simulink model "TRN_KAISIM"  (R2022a)
settings: Solver=FixedStepAuto  StartTime=0.0  StopTime=300  FixedStep=0.04  RelTol=1e-3
PreLoadFcn:
  | load('BusStructureTRNsensor.mat');
  | load('BusStructureTRN.mat');
InitFcn:
  | load('BusStructureTRNsensor.mat');
  | load('BusStructureTRN.mat');
undefined symbols (not defined in the file or in its folder): Altitude_INS, Latitude_INS, Longitude_INS, residual, Result_Prev, TimeTag_Prev, TRN, TRNlib
libraries: simulink_extras x18, sharedtransform x3
(part 2 of 4)

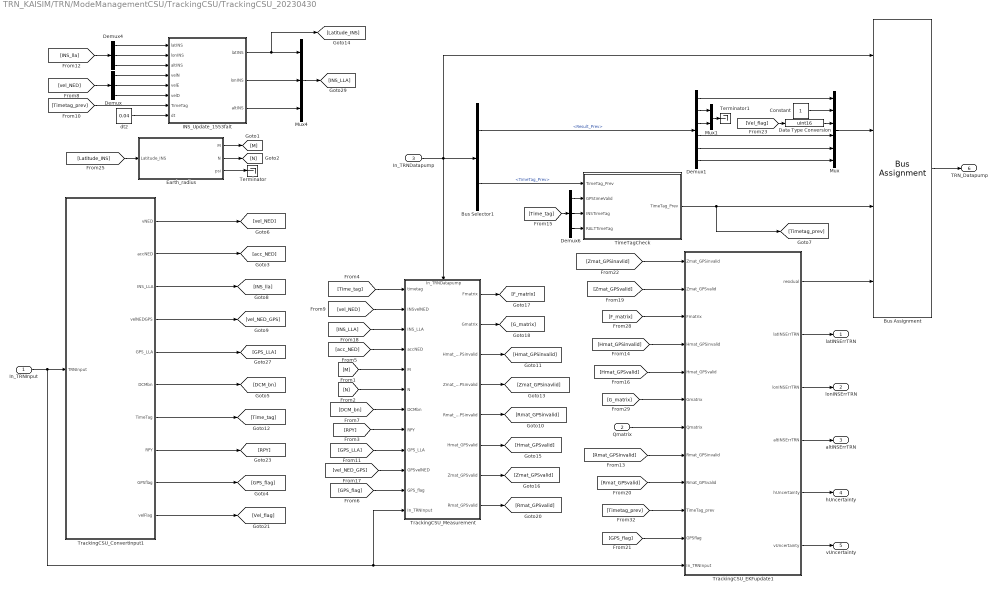
== system TRN_KAISIM/TRN/ModeManagementCSU/TrackingCSU/TrackingCSU_20230430 ==
  In_TRNInput : Inport  OutDataTypeStr=Bus: TRNInput
  Qmatrix : Inport  Port=2
  In_TRNDatapump : Inport  Port=3  OutDataTypeStr=Bus: TRNDatapump  PortDimensions=1
  Bus Assignment : BusAssignment  AssignedSignals=Result_Prev,TimeTag_Prev,residual
  Bus Selector1 : BusSelector  OutputSignals=Result_Prev,TimeTag_Prev
  Constant : Constant  OutDataTypeStr=uint16
  Data Type Conversion : DataTypeConversion  OutDataTypeStr=uint16  SaturateOnIntegerOverflow=off  RndMeth=Floor
  Demux : Demux  Outputs=3
  Demux1 : Demux  Outputs=6
  Demux4 : Demux  Outputs=3
  Demux6 : Demux  Outputs=3
  Earth_radius : MATLAB Function  TreatAsAtomicUnit=on
      settings: RTWSystemCode=Nonreusable function  RTWFcnNameOpts=Use subsystem name
  INS_Update_1553falt : MATLAB Function  TreatAsAtomicUnit=on
      settings: RTWSystemCode=Nonreusable function  RTWFcnNameOpts=Use subsystem name
  Mux : Mux  Inputs=6
  Mux1 : Mux  Inputs=2
  Mux4 : Mux  Inputs=3
  Terminator : Terminator
  Terminator1 : Terminator
  TimeTagCheck : MATLAB Function  TreatAsAtomicUnit=on
      settings: RTWSystemCode=Nonreusable function  RTWFcnNameOpts=Use subsystem name
  TrackingCSU_ConvertInput1 : Subsystem  TreatAsAtomicUnit=on
      settings: RTWSystemCode=Nonreusable function  RTWFcnNameOpts=Use subsystem name
  TrackingCSU_EKFupdate1 : Subsystem  TreatAsAtomicUnit=on
      settings: RTWSystemCode=Nonreusable function  RTWFcnNameOpts=Use subsystem name
  TrackingCSU_Measurement : Subsystem  TreatAsAtomicUnit=on
      settings: RTWSystemCode=Nonreusable function  RTWFcnNameOpts=Use subsystem name  PortSchema="{\"entries\":[{\"content\":{\"sides\":[{\"content\":{\"connectorIds\":[\"In1\",\"In2\",\"In3\",\"In4\",\"In5\",\"In6\",\"In7\",\"In8\",\"In9\",\"In10\",\"In11\",\"In12\"]},\"type\":\"ConnectorPlacement.EquallySpacedRectSide\",\"uuid\":\"284c5e42-61c1-4616-966e-143f60f46571\"},{\"content\":{\"connectorIds\":[\"Out1\",\"Out2\",\"Out3\",\"Out4\",\"Out5\",\"Out6\",\"Out7\",\"Out8\"],\"side\":\"RIGHT\"},\"type\":\"ConnectorPlacement.EquallySpacedRectSide\",\"uuid\":\"be5b0b09-4e69-4cdf-8a94-a8639994cbf9\"},{\"content\":{\"connectorIds\":[\"In13\"],\"side\":\"TOP\"},\"type\":\"ConnectorPlacement.EquallySpacedRectSide\",\"uuid\":\"f7fbee8b-afe7-4fec-8c40-a5bd5e14374e\"},{\"content\":{\"connectorIds\":[],\"side\":\"BOTTOM\"},\"type\":\"ConnectorPlacement.EquallySpacedRectSide\",\"uuid\":\"9a503e43-aaca-441a-ab76-b52386228bc3\"}]},\"type\":\"ConnectorPlacement.EquallySpacedConnector\",\"uuid\":\"1b32203e-baad-4c49-8c24-20b6a9ecb4b9\"}],\"packageUris\":[\"http://schema.mathworks.com/mf0/Connector/R2020b\"],\"version\":\"1.0\"}"
  dt2 : Constant  Value=0.04  OutDataTypeStr=double
  latINSErrTRN : Outport
  lonINSErrTRN : Outport  Port=2
  altINSErrTRN : Outport  Port=3
  hUncertainty : Outport  Port=4
  vUncertainty : Outport  Port=5
  TRN_Datapump : Outport  Port=6  OutDataTypeStr=Bus: TRNDatapump
  wires:
  Mux4/1 -> [INS_LLA]
  Demux/3 -> INS_Update_1553falt/6(velD)
  Demux/1 -> INS_Update_1553falt/4(velN)
  Demux/2 -> INS_Update_1553falt/5(velE)
  dt2/1 -> INS_Update_1553falt/8(dt)
  Bus Selector1/2 -> TimeTagCheck/1("TimeTag_Prev ")  "<TimeTag_Prev>"
  In_TRNDatapump/1 -> TrackingCSU_Measurement/13(In_TRNDatapump), Bus Selector1/1, Bus Assignment/1
  INS_Update_1553falt/3(altINS) -> Mux4/3
  In_TRNInput/1 -> TrackingCSU_ConvertInput1/1(TRNInput), TrackingCSU_EKFupdate1/12(In_TRNInput), TrackingCSU_Measurement/12(In_TRNInput)
  INS_Update_1553falt/1(latINS) -> [Latitude_INS], Mux4/1
  INS_Update_1553falt/2(lonINS) -> Mux4/2
  TrackingCSU_ConvertInput1/2(accNED) -> [acc_NED]
  TrackingCSU_ConvertInput1/6(DCMbn) -> [DCM_bn]
  TrackingCSU_ConvertInput1/1(vNED) -> [vel_NED]
  [vel_NED] -> Demux/1
  [Timetag_prev] -> INS_Update_1553falt/7(TimeTag)
  [INS_lla] -> Demux4/1
  Demux4/2 -> INS_Update_1553falt/2("lonINS ")
  Demux4/1 -> INS_Update_1553falt/1("latINS ")
  Demux4/3 -> INS_Update_1553falt/3("altINS ")
  TrackingCSU_ConvertInput1/4(velNEDGPS) -> [vel_NED_GPS]
  [Time_tag] -> Demux6/1
  Demux6/1 -> TimeTagCheck/2(GPStimeValid)
  Demux6/2 -> TimeTagCheck/3(INSTimeTag)
  Demux6/3 -> TimeTagCheck/4(RALTTimeTag)
  TrackingCSU_Measurement/1(Fmatrix) -> [F_matrix]
  TrackingCSU_Measurement/2(Gmatrix) -> [G_matrix]
  [Zmat_GPSinavlid] -> TrackingCSU_EKFupdate1/1(Zmat_GPSinvalid)
  [Latitude_INS] -> Earth_radius/1(Latitude_INS)
  Earth_radius/1(M) -> [M]
  Earth_radius/2(N) -> [N]
  TrackingCSU_ConvertInput1/5(GPS_LLA) -> [GPS_LLA]
  TrackingCSU_ConvertInput1/8(RPY) -> [RPY]
  TimeTagCheck/1(TimeTag_Prev) -> [Timetag_prev], Bus Assignment/3
  TrackingCSU_ConvertInput1/9(GPSflag) -> [GPS_flag]
  TrackingCSU_ConvertInput1/7(TimeTag) -> [Time_tag]
  TrackingCSU_ConvertInput1/3(INS_LLA) -> [INS_lla]
  Earth_radius/3(psi) -> Terminator/1
  TrackingCSU_Measurement/3(Hmat_GPSinvalid) -> [Hmat_GPSinvalid]
  TrackingCSU_Measurement/4(Zmat_GPSinvalid) -> [Zmat_GPSinavlid]
  TrackingCSU_Measurement/5(Rmat_GPSinvalid) -> [Rmat_GPSinvalid]
  TrackingCSU_Measurement/6(Hmat_GPSvalid) -> [Hmat_GPSvalid]
  TrackingCSU_Measurement/7(Zmat_GPSvalid) -> [Zmat_GPSvalid]
  TrackingCSU_Measurement/8(Rmat_GPSvalid) -> [Rmat_GPSvalid]
  [GPS_flag] -> TrackingCSU_EKFupdate1/11(GPSflag)
  [Rmat_GPSvalid] -> TrackingCSU_EKFupdate1/9(Rmat_GPSvalid)
  [Rmat_GPSinvalid] -> TrackingCSU_EKFupdate1/8(Rmat_GPSinvalid)
  Qmatrix/1 -> TrackingCSU_EKFupdate1/7(Qmatrix)
  [G_matrix] -> TrackingCSU_EKFupdate1/6(Gmatrix)
  [Hmat_GPSvalid] -> TrackingCSU_EKFupdate1/5(Hmat_GPSvalid)
  [Hmat_GPSinvalid] -> TrackingCSU_EKFupdate1/4(Hmat_GPSinvalid)
  [F_matrix] -> TrackingCSU_EKFupdate1/3(Fmatrix)
  [Zmat_GPSvalid] -> TrackingCSU_EKFupdate1/2(Zmat_GPSvalid)
  TrackingCSU_EKFupdate1/2(latINSErrTRN) -> latINSErrTRN/1
  TrackingCSU_EKFupdate1/3(lonINSErrTRN) -> lonINSErrTRN/1
  TrackingCSU_EKFupdate1/4(altINSErrTRN) -> altINSErrTRN/1
  TrackingCSU_EKFupdate1/5(hUncertainty) -> hUncertainty/1
  TrackingCSU_EKFupdate1/6(vUncertainty) -> vUncertainty/1
  [Timetag_prev] -> TrackingCSU_EKFupdate1/10(TimeTag_prev)
  [GPS_LLA] -> TrackingCSU_Measurement/9(GPS_LLA)
  [vel_NED_GPS] -> TrackingCSU_Measurement/10(GPSvelNED)
  [GPS_flag] -> TrackingCSU_Measurement/11(GPS_flag)
  [Time_tag] -> TrackingCSU_Measurement/1(timetag)
  [INS_LLA] -> TrackingCSU_Measurement/3(INS_LLA)
  [acc_NED] -> TrackingCSU_Measurement/4(accNED)
  [DCM_bn] -> TrackingCSU_Measurement/7(DCMbn)
  [RPY] -> TrackingCSU_Measurement/8(RPY)
  [M] -> TrackingCSU_Measurement/5(M)
  [N] -> TrackingCSU_Measurement/6(N)
  [vel_NED] -> TrackingCSU_Measurement/2(INSvelNED)
  Bus Assignment/1 -> TRN_Datapump/1
  Mux/1 -> Bus Assignment/2
  Demux1/1 -> Mux/1
  Demux1/5 -> Mux/5
  Demux1/6 -> Mux/6
  TrackingCSU_ConvertInput1/10(velFlag) -> [Vel_flag]
  [Vel_flag] -> Data Type Conversion/1
  Data Type Conversion/1 -> Mux/3
  Constant/1 -> Mux/2
  Demux1/4 -> Mux/4
  Demux1/3 -> Mux1/2
  Demux1/2 -> Mux1/1
  Mux1/1 -> Terminator1/1
  Bus Selector1/1 -> Demux1/1  "<Result_Prev>"
  TrackingCSU_EKFupdate1/1(residual) -> Bus Assignment/4

== system TRN_KAISIM/TRN/TRN_visualization/Subsystem ==
  In1 : Inport
  In2 : Inport  Port=2
  In3 : Inport  Port=3
  In4 : Inport  Port=4
  In5 : Inport  Port=5
  In6 : Inport  Port=6
  Gain2 : Gain  Gain=111000
  Gain3 : Gain  Gain=91170
  MATLAB Function1 : MATLAB Function  TreatAsAtomicUnit=on
  Sum : Sum  Inputs=|+-
  Sum1 : Sum  Inputs=|+-
  Sum2 : Sum  Inputs=|+-
  Terrain_Level_big4 : MATLAB Function  TreatAsAtomicUnit=on
  TRN Position Error Horizon : Outport
  TRN Position Error Vertical : Outport  Port=2
  Roughness : Outport  Port=3
  wires:
  Sum1/1 -> Gain3/1
  In1/1 -> Terrain_Level_big4/1(Lat), Sum/1
  In3/1 -> Terrain_Level_big4/2(Lon), Sum1/1
  Terrain_Level_big4/1(R) -> Roughness/1
  Gain2/1 -> MATLAB Function1/1(y)  "LatErr"
  Gain3/1 -> MATLAB Function1/2(x)  "LonErr"
  Sum2/1 -> TRN Position Error Vertical/1
  Sum/1 -> Gain2/1
  In4/1 -> Sum1/2
  In2/1 -> Sum/2
  In6/1 -> Sum2/2
  In5/1 -> Sum2/1
  MATLAB Function1/1(a) -> TRN Position Error Horizon/1

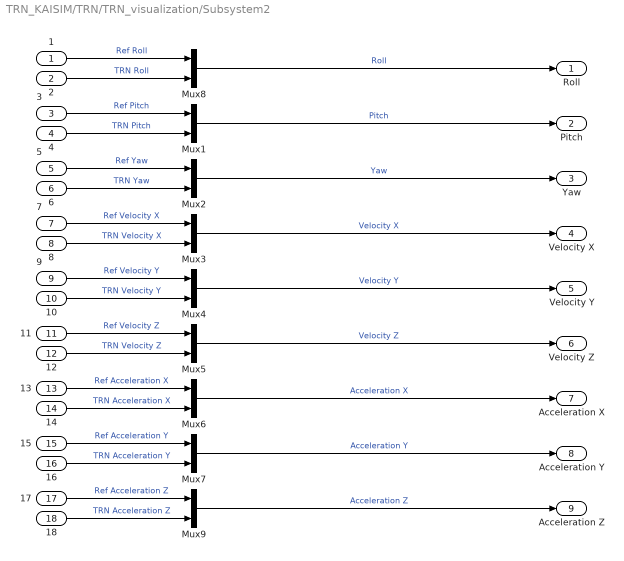
== system TRN_KAISIM/TRN/TRN_visualization/Subsystem2 ==
  1 : Inport
  2 : Inport  Port=2
  3 : Inport  Port=3
  4 : Inport  Port=4
  5 : Inport  Port=5
  6 : Inport  Port=6
  7 : Inport  Port=7
  8 : Inport  Port=8
  9 : Inport  Port=9
  10 : Inport  Port=10
  11 : Inport  Port=11
  12 : Inport  Port=12
  13 : Inport  Port=13
  14 : Inport  Port=14
  15 : Inport  Port=15
  16 : Inport  Port=16
  17 : Inport  Port=17
  18 : Inport  Port=18
  Mux{1..9} (9 alike) : Mux  Inputs=2
  Roll : Outport
  Pitch : Outport  Port=2
  Yaw : Outport  Port=3
  Velocity X : Outport  Port=4
  Velocity Y : Outport  Port=5
  Velocity Z : Outport  Port=6
  Acceleration X : Outport  Port=7
  Acceleration Y : Outport  Port=8
  Acceleration Z : Outport  Port=9
  wires:
  3/1 -> Mux1/1  "Ref Pitch"
  12/1 -> Mux5/2  "TRN Velocity Z"
  10/1 -> Mux4/2  "TRN Velocity Y"
  Mux9/1 -> Acceleration Z/1  "Acceleration Z"
  Mux8/1 -> Roll/1  "Roll"
  9/1 -> Mux4/1  "Ref Velocity Y"
  8/1 -> Mux3/2  "TRN Velocity X"
  5/1 -> Mux2/1  "Ref Yaw"
  Mux4/1 -> Velocity Y/1  "Velocity Y"
  1/1 -> Mux8/1  "Ref Roll"
  Mux6/1 -> Acceleration X/1  "Acceleration X"
  Mux7/1 -> Acceleration Y/1  "Acceleration Y"
  4/1 -> Mux1/2  "TRN Pitch"
  11/1 -> Mux5/1  "Ref Velocity Z"
  16/1 -> Mux7/2  "TRN Acceleration Y"
  Mux3/1 -> Velocity X/1  "Velocity X"
  Mux2/1 -> Yaw/1  "Yaw"
  2/1 -> Mux8/2  "TRN Roll"
  6/1 -> Mux2/2  "TRN Yaw"
  7/1 -> Mux3/1  "Ref Velocity X"
  Mux5/1 -> Velocity Z/1  "Velocity Z"
  Mux1/1 -> Pitch/1  "Pitch"
  15/1 -> Mux7/1  "Ref Acceleration Y"
  14/1 -> Mux6/2  "TRN Acceleration X"
  17/1 -> Mux9/1  "Ref Acceleration Z"
  18/1 -> Mux9/2  "TRN Acceleration Z"
  13/1 -> Mux6/1  "Ref Acceleration X"

== system TRN_KAISIM/TRN/TRN_visualization/Subsystem3 ==
  In1 : Inport
  In2 : Inport  Port=2
  In3 : Inport  Port=3
  In4 : Inport  Port=4
  In5 : Inport  Port=5
  In6 : Inport  Port=6
  Gain2 : Gain  Gain=111000
  Gain3 : Gain  Gain=91170
  MATLAB Function1 : MATLAB Function  TreatAsAtomicUnit=on
  Sum : Sum  Inputs=|+-
  Sum1 : Sum  Inputs=|+-
  Sum2 : Sum  Inputs=|+-
  Terrain_Level : MATLAB Function  TreatAsAtomicUnit=on
  TRN Position Error Horizon : Outport
  TRN Position Error Vertical : Outport  Port=2
  Roughness : Outport  Port=3
  wires:
  Sum1/1 -> Gain3/1
  In1/1 -> Terrain_Level/1(Lat), Sum/1
  In3/1 -> Terrain_Level/2(Lon), Sum1/1
  Terrain_Level/1(R) -> Roughness/1
  Gain2/1 -> MATLAB Function1/1(y)  "LatErr"
  Gain3/1 -> MATLAB Function1/2(x)  "LonErr"
  Sum2/1 -> TRN Position Error Vertical/1
  Sum/1 -> Gain2/1
  In4/1 -> Sum1/2
  In2/1 -> Sum/2
  In6/1 -> Sum2/2
  In5/1 -> Sum2/1
  MATLAB Function1/1(a) -> TRN Position Error Horizon/1

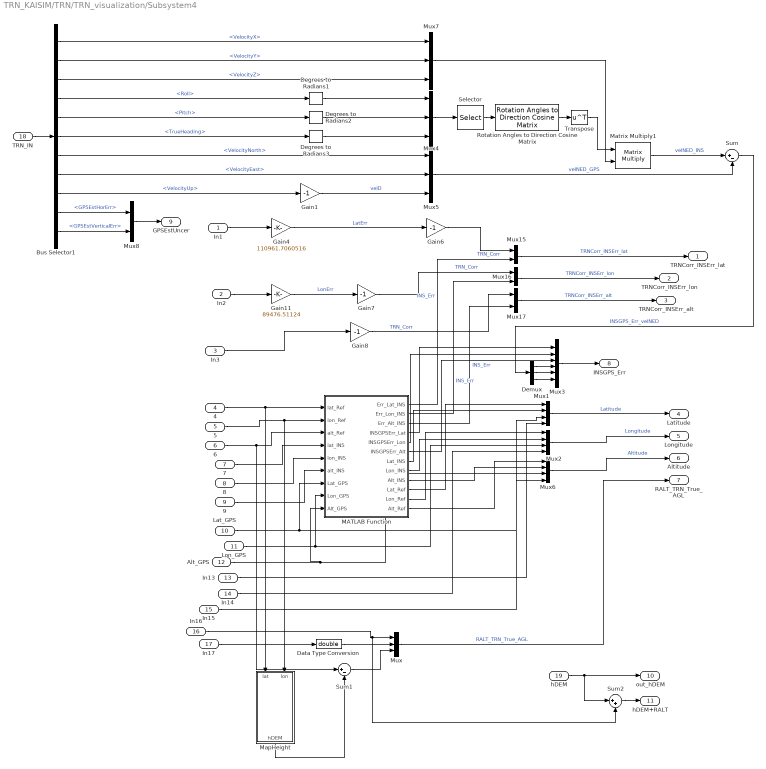
== system TRN_KAISIM/TRN/TRN_visualization/Subsystem4 ==
  In1 : Inport
  In2 : Inport  Port=2
  In3 : Inport  Port=3
  4 : Inport  Port=4
  5 : Inport  Port=5
  6 : Inport  Port=6
  7 : Inport  Port=7
  8 : Inport  Port=8
  9 : Inport  Port=9
  Lat_GPS : Inport  Port=10
  Lon_GPS : Inport  Port=11
  Alt_GPS : Inport  Port=12
  In13 : Inport  Port=13
  In14 : Inport  Port=14
  In15 : Inport  Port=15
  In16 : Inport  Port=16
  In17 : Inport  Port=17
  TRN_IN : Inport  Port=18
  hDEM : Inport  Port=19
  Bus Selector1 : BusSelector  OutputSignals=VelocityX,VelocityY,VelocityZ,Roll,Pitch,TrueHeading,VelocityNorth,VelocityEast,VelocityUp,GPSEstHorErr,GPSEstVerticalErr
  Data Type Conversion : DataTypeConversion  OutDataTypeStr=double  SaturateOnIntegerOverflow=off  RndMeth=Floor
  Degrees to Radians1 : simulink_extras/Transformations/Degrees to Radians
  Degrees to Radians2 : simulink_extras/Transformations/Degrees to Radians
  Degrees to Radians3 : simulink_extras/Transformations/Degrees to Radians
  Demux : Demux  Outputs=3
  Gain{1,6..8} (4 alike) : Gain  Gain=-1
  Gain11 : Gain  Gain=89476.51124
  Gain4 : Gain  Gain=110961.7060516
  MATLAB Function : MATLAB Function  TreatAsAtomicUnit=on
  MapHeight : MATLAB Function  TreatAsAtomicUnit=on
  Matrix Multiply1 : Product  Multiplication=Matrix(*)
  Mux{,4..5,7} (4 alike) : Mux  Inputs=3
  Mux1 : Mux
  Mux{8,15..17} (4 alike) : Mux  Inputs=2
  Mux2 : Mux
  Mux3 : Mux  Inputs=6
  Mux6 : Mux
  Rotation Angles to Direction Cosine Matrix : sharedtransform/Rotation Angles to Direction Cosine Matrix  rotationOrder=ZYX  aMode=aMode
      settings: SourceProductBaseCode=AE,PW,DR,MT,VE
  Selector : Selector  InputPortWidth=3  IndexOptions=Index vector (dialog)  Indices=[3 2 1]  OutputSizes=1
  Sum : Sum  Inputs=|+-
  Sum1 : Sum  Inputs=|+-
  Sum2 : Sum  Inputs=|++
  Transpose : Math  Operator=transpose  SignedPower=on
  TRNCorr_INSErr_lat : Outport
  TRNCorr_INSErr_lon : Outport  Port=2
  TRNCorr_INSErr_alt : Outport  Port=3
  Latitude : Outport  Port=4
  Longitude : Outport  Port=5
  Altitude : Outport  Port=6
  RALT_TRN_True_AGL : Outport  Port=7
  INSGPS_Err : Outport  Port=8
  GPSEstUncer : Outport  Port=9
  out_hDEM : Outport  Port=10
  hDEM+RALT : Outport  Port=11
  wires:
  7/1 -> MATLAB Function/4(lat_INS)
  MATLAB Function/10(Lat_Ref) -> Mux1/1
  Gain8/1 -> Mux17/1  "TRN_Corr"
  MATLAB Function/7(Lat_INS) -> Mux1/2
  MATLAB Function/8(Lon_INS) -> Mux2/2
  MATLAB Function/3(Err_Alt_INS) -> Mux17/2  "INS_Err"
  In13/1 -> Mux1/4
  Gain7/1 -> Mux16/1  "TRN_Corr"
  Mux1/1 -> Latitude/1  "Latitude"
  MATLAB Function/1(Err_Lat_INS) -> Mux15/2  "INS_Err"
  MATLAB Function/12(Alt_Ref) -> Mux6/1
  4/1 -> MapHeight/1(lat), MATLAB Function/1(lat_Ref)
  Gain11/1 -> Gain7/1  "LonErr"
  Gain6/1 -> Mux15/1  "TRN_Corr"
  MATLAB Function/9(Alt_INS) -> Mux6/2
  MATLAB Function/2(Err_Lon_INS) -> Mux16/2  "INS_Err"
  Mux17/1 -> TRNCorr_INSErr_alt/1  "TRNCorr_INSErr_alt"
  Gain4/1 -> Gain6/1  "LatErr"
  MATLAB Function/11(Lon_Ref) -> Mux2/1
  Lat_GPS/1 -> MATLAB Function/7(Lat_GPS), Mux1/3
  Mux2/1 -> Longitude/1  "Longitude"
  In3/1 -> Gain8/1
  Data Type Conversion/1 -> Mux/2
  8/1 -> MATLAB Function/5(lon_INS)
  Mux/1 -> RALT_TRN_True_AGL/1  "RALT_TRN_True_AGL"
  In17/1 -> Data Type Conversion/1
  9/1 -> MATLAB Function/6(alt_INS)
  Lon_GPS/1 -> MATLAB Function/8(Lon_GPS), Mux2/3
  Alt_GPS/1 -> MATLAB Function/9(Alt_GPS), Mux6/3
  In2/1 -> Gain11/1
  Mux16/1 -> TRNCorr_INSErr_lon/1  "TRNCorr_INSErr_lon"
  Mux6/1 -> Altitude/1  "Altitude"
  In1/1 -> Gain4/1
  In15/1 -> Mux6/4
  In14/1 -> Mux2/4
  6/1 -> Sum1/1, MATLAB Function/3(alt_Ref)
  5/1 -> MapHeight/2(lon), MATLAB Function/2(lon_Ref)
  Mux15/1 -> TRNCorr_INSErr_lat/1  "TRNCorr_INSErr_lat"
  MATLAB Function/5(INSGPSErr_Lon) -> Mux3/2
  MATLAB Function/4(INSGPSErr_Lat) -> Mux3/1
  MATLAB Function/6(INSGPSErr_Alt) -> Mux3/3
  Mux3/1 -> INSGPS_Err/1
  Mux7/1 -> Matrix Multiply1/2
  Degrees to Radians3/1 -> Mux4/3
  Degrees to Radians1/1 -> Mux4/1
  Bus Selector1/4 -> Degrees to Radians1/1  "<Roll>"
  Bus Selector1/6 -> Degrees to Radians3/1  "<TrueHeading>"
  Matrix Multiply1/1 -> Sum/1  "velNED_INS"
  Bus Selector1/5 -> Degrees to Radians2/1  "<Pitch>"
  Degrees to Radians2/1 -> Mux4/2
  Bus Selector1/2 -> Mux7/2  "<VelocityY>"
  Bus Selector1/1 -> Mux7/1  "<VelocityX>"
  Mux4/1 -> Selector/1
  Transpose/1 -> Matrix Multiply1/1
  Bus Selector1/3 -> Mux7/3  "<VelocityZ>"
  TRN_IN/1 -> Bus Selector1/1
  Rotation Angles to Direction Cosine Matrix/1 -> Transpose/1
  Selector/1 -> Rotation Angles to Direction Cosine Matrix/1
  Bus Selector1/7 -> Mux5/1  "<VelocityNorth>"
  Bus Selector1/8 -> Mux5/2  "<VelocityEast>"
  Bus Selector1/9 -> Gain1/1  "<VelocityUp>"
  Gain1/1 -> Mux5/3  "velD"
  Mux5/1 -> Sum/2  "velNED_GPS"
  Demux/1 -> Mux3/4
  Demux/2 -> Mux3/5
  Demux/3 -> Mux3/6
  Sum/1 -> Demux/1  "INSGPS_Err_velNED"
  Bus Selector1/10 -> Mux8/1  "<GPSEstHorErr>"
  Bus Selector1/11 -> Mux8/2  "<GPSEstVerticalErr>"
  Mux8/1 -> GPSEstUncer/1
  MapHeight/1(hDEM) -> Sum1/2
  Sum1/1 -> Mux/3
  In16/1 -> Sum2/2, Mux/1
  hDEM/1 -> out_hDEM/1, Sum2/1
  Sum2/1 -> hDEM+RALT/1

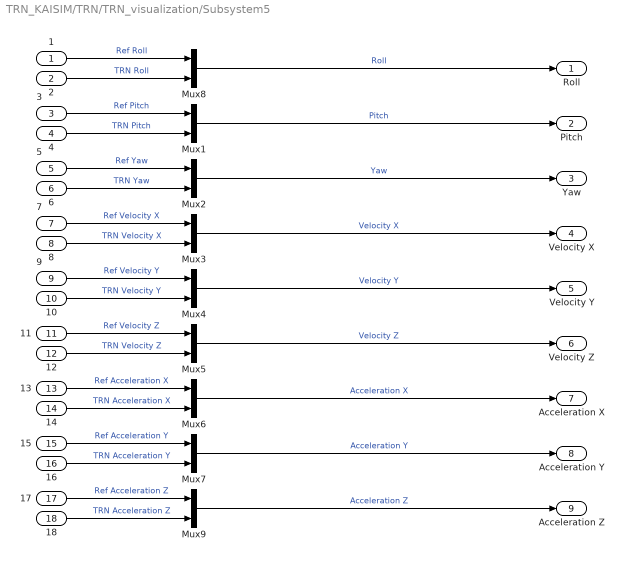
== system TRN_KAISIM/TRN/TRN_visualization/Subsystem5 ==
  1 : Inport
  2 : Inport  Port=2
  3 : Inport  Port=3
  4 : Inport  Port=4
  5 : Inport  Port=5
  6 : Inport  Port=6
  7 : Inport  Port=7
  8 : Inport  Port=8
  9 : Inport  Port=9
  10 : Inport  Port=10
  11 : Inport  Port=11
  12 : Inport  Port=12
  13 : Inport  Port=13
  14 : Inport  Port=14
  15 : Inport  Port=15
  16 : Inport  Port=16
  17 : Inport  Port=17
  18 : Inport  Port=18
  Mux{1..9} (9 alike) : Mux  Inputs=2
  Roll : Outport
  Pitch : Outport  Port=2
  Yaw : Outport  Port=3
  Velocity X : Outport  Port=4
  Velocity Y : Outport  Port=5
  Velocity Z : Outport  Port=6
  Acceleration X : Outport  Port=7
  Acceleration Y : Outport  Port=8
  Acceleration Z : Outport  Port=9
  wires:
  3/1 -> Mux1/1  "Ref Pitch"
  12/1 -> Mux5/2  "TRN Velocity Z"
  10/1 -> Mux4/2  "TRN Velocity Y"
  Mux9/1 -> Acceleration Z/1  "Acceleration Z"
  Mux8/1 -> Roll/1  "Roll"
  9/1 -> Mux4/1  "Ref Velocity Y"
  8/1 -> Mux3/2  "TRN Velocity X"
  5/1 -> Mux2/1  "Ref Yaw"
  Mux4/1 -> Velocity Y/1  "Velocity Y"
  1/1 -> Mux8/1  "Ref Roll"
  Mux6/1 -> Acceleration X/1  "Acceleration X"
  Mux7/1 -> Acceleration Y/1  "Acceleration Y"
  4/1 -> Mux1/2  "TRN Pitch"
  11/1 -> Mux5/1  "Ref Velocity Z"
  16/1 -> Mux7/2  "TRN Acceleration Y"
  Mux3/1 -> Velocity X/1  "Velocity X"
  Mux2/1 -> Yaw/1  "Yaw"
  2/1 -> Mux8/2  "TRN Roll"
  6/1 -> Mux2/2  "TRN Yaw"
  7/1 -> Mux3/1  "Ref Velocity X"
  Mux5/1 -> Velocity Z/1  "Velocity Z"
  Mux1/1 -> Pitch/1  "Pitch"
  15/1 -> Mux7/1  "Ref Acceleration Y"
  14/1 -> Mux6/2  "TRN Acceleration X"
  17/1 -> Mux9/1  "Ref Acceleration Z"
  18/1 -> Mux9/2  "TRN Acceleration Z"
  13/1 -> Mux6/1  "Ref Acceleration X"

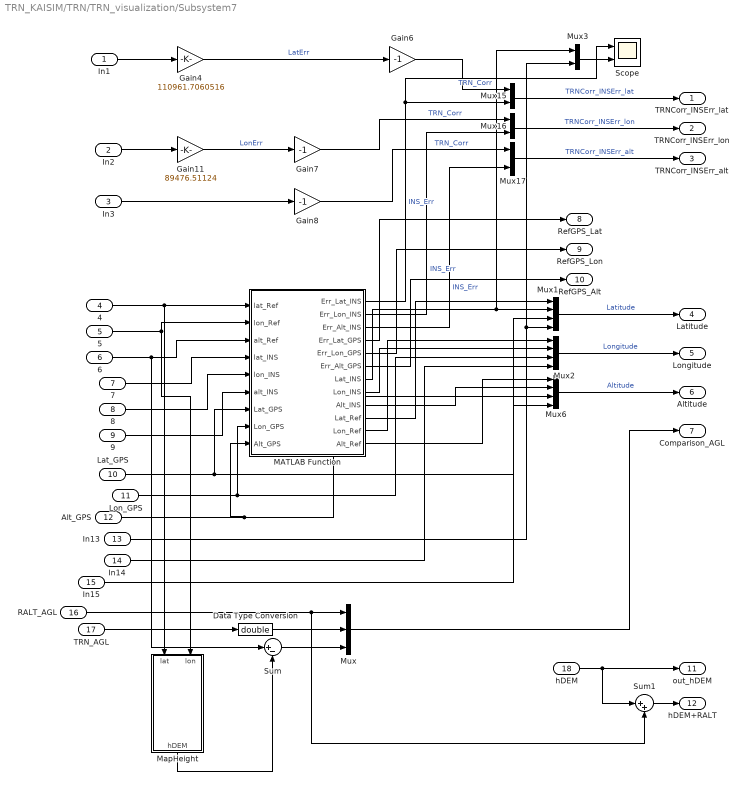
== system TRN_KAISIM/TRN/TRN_visualization/Subsystem7 ==
  In1 : Inport
  In2 : Inport  Port=2
  In3 : Inport  Port=3
  4 : Inport  Port=4
  5 : Inport  Port=5
  6 : Inport  Port=6
  7 : Inport  Port=7
  8 : Inport  Port=8
  9 : Inport  Port=9
  Lat_GPS : Inport  Port=10
  Lon_GPS : Inport  Port=11
  Alt_GPS : Inport  Port=12
  In13 : Inport  Port=13
  In14 : Inport  Port=14
  In15 : Inport  Port=15
  RALT_AGL : Inport  Port=16
  TRN_AGL : Inport  Port=17
  hDEM : Inport  Port=18
  Data Type Conversion : DataTypeConversion  OutDataTypeStr=double  SaturateOnIntegerOverflow=off  RndMeth=Floor
  Gain11 : Gain  Gain=89476.51124
  Gain4 : Gain  Gain=110961.7060516
  Gain6 : Gain  Gain=-1
  Gain7 : Gain  Gain=-1
  Gain8 : Gain  Gain=-1
  MATLAB Function : MATLAB Function  TreatAsAtomicUnit=on
  MapHeight : MATLAB Function  TreatAsAtomicUnit=on
  Mux : Mux  Inputs=3
  Mux1 : Mux
  Mux{3,15..17} (4 alike) : Mux  Inputs=2
  Mux2 : Mux
  Mux6 : Mux
  Scope : Scope  NumInputPorts=2
  Sum : Sum  Inputs=|+-
  Sum1 : Sum  Inputs=|++
  TRNCorr_INSErr_lat : Outport
  TRNCorr_INSErr_lon : Outport  Port=2
  TRNCorr_INSErr_alt : Outport  Port=3
  Latitude : Outport  Port=4
  Longitude : Outport  Port=5
  Altitude : Outport  Port=6
  Comparison_AGL : Outport  Port=7
  RefGPS_Lat : Outport  Port=8
  RefGPS_Lon : Outport  Port=9
  RefGPS_Alt : Outport  Port=10
  out_hDEM : Outport  Port=11
  hDEM+RALT : Outport  Port=12
  wires:
  Mux15/1 -> TRNCorr_INSErr_lat/1  "TRNCorr_INSErr_lat"
  5/1 -> MapHeight/2(lon), MATLAB Function/2(lon_Ref)
  6/1 -> Sum/1, MATLAB Function/3(alt_Ref)
  In14/1 -> Mux2/4
  In15/1 -> Mux6/4
  In1/1 -> Gain4/1
  Mux6/1 -> Altitude/1  "Altitude"
  Mux16/1 -> TRNCorr_INSErr_lon/1  "TRNCorr_INSErr_lon"
  In2/1 -> Gain11/1
  Alt_GPS/1 -> Mux6/3, MATLAB Function/9(Alt_GPS)
  Lon_GPS/1 -> Mux2/3, MATLAB Function/8(Lon_GPS)
  9/1 -> MATLAB Function/6(alt_INS)
  RALT_AGL/1 -> Sum1/2, Mux/1
  TRN_AGL/1 -> Data Type Conversion/1
  Mux/1 -> Comparison_AGL/1
  8/1 -> MATLAB Function/5(lon_INS)
  Data Type Conversion/1 -> Mux/2
  In3/1 -> Gain8/1
  Mux2/1 -> Longitude/1  "Longitude"
  Lat_GPS/1 -> Mux1/3, MATLAB Function/7(Lat_GPS)
  MATLAB Function/11(Lon_Ref) -> Mux2/1
  Gain4/1 -> Gain6/1  "LatErr"
  Mux17/1 -> TRNCorr_INSErr_alt/1  "TRNCorr_INSErr_alt"
  MATLAB Function/2(Err_Lon_INS) -> Mux16/2  "INS_Err"
  MATLAB Function/9(Alt_INS) -> Mux6/2
  Gain6/1 -> Mux15/1  "TRN_Corr"
  Gain11/1 -> Gain7/1  "LonErr"
  4/1 -> MATLAB Function/1(lat_Ref), MapHeight/1(lat)
  MATLAB Function/12(Alt_Ref) -> Mux6/1
  MATLAB Function/1(Err_Lat_INS) -> Scope/1, Mux15/2  "INS_Err"
  Mux1/1 -> Latitude/1  "Latitude"
  Gain7/1 -> Mux16/1  "TRN_Corr"
  In13/1 -> Mux3/2, Mux1/4
  MATLAB Function/3(Err_Alt_INS) -> Mux17/2  "INS_Err"
  MATLAB Function/8(Lon_INS) -> Mux2/2
  MATLAB Function/7(Lat_INS) -> Mux3/1, Mux1/2
  Gain8/1 -> Mux17/1  "TRN_Corr"
  MATLAB Function/10(Lat_Ref) -> Mux1/1
  7/1 -> MATLAB Function/4(lat_INS)
  MATLAB Function/4(Err_Lat_GPS) -> RefGPS_Lat/1
  MATLAB Function/5(Err_Lon_GPS) -> RefGPS_Lon/1
  MATLAB Function/6(Err_Alt_GPS) -> RefGPS_Alt/1
  Sum/1 -> Mux/3
  MapHeight/1(hDEM) -> Sum/2
  hDEM/1 -> out_hDEM/1, Sum1/1
  Sum1/1 -> hDEM+RALT/1
  Mux3/1 -> Scope/2

== system TRN_KAISIM/TRN/ModeManagementCSU/AcquisitionCSU/AcquisitionCSU/ConvertTRNInput ==
  TRNInput : Inport  OutDataTypeStr=Bus: TRNInput
  Bus Selector1 : BusSelector  OutputSignals=Latitude_INS,Longitude_INS,Altitude_INS,RALTAltitude,GPSDataNotValid,Latitude_GPS,Longitude_GPS,Altitude_GPS,INSDataNotValid,FigureofMerit
  Degrees to Radians{1..2,4..5} (4 alike) : simulink_extras/Transformations/Degrees to Radians
  latINS : Outport  VectorParamsAs1DForOutWhenUnconnected=off
  lonINS : Outport  Port=2  VectorParamsAs1DForOutWhenUnconnected=off
  altINS : Outport  Port=3  VectorParamsAs1DForOutWhenUnconnected=off
  altRALT : Outport  Port=4  VectorParamsAs1DForOutWhenUnconnected=off
  latGPS : Outport  Port=5  VectorParamsAs1DForOutWhenUnconnected=off
  lonGPS : Outport  Port=6  VectorParamsAs1DForOutWhenUnconnected=off
  altGPS : Outport  Port=7  VectorParamsAs1DForOutWhenUnconnected=off
  GPSDataNotValid : Outport  Port=8  VectorParamsAs1DForOutWhenUnconnected=off
  INSDataNotValid : Outport  Port=9  VectorParamsAs1DForOutWhenUnconnected=off
  FigureofMerit : Outport  Port=10  VectorParamsAs1DForOutWhenUnconnected=off
  wires:
  Bus Selector1/9 -> INSDataNotValid/1  "<INSDataNotValid>"
  Bus Selector1/2 -> Degrees to Radians4/1  "<Longitude_INS>"
  Bus Selector1/1 -> Degrees to Radians5/1  "<Latitude_INS>"
  Bus Selector1/4 -> altRALT/1  "<RALTAltitude>"
  Degrees to Radians4/1 -> lonINS/1
  Degrees to Radians5/1 -> latINS/1
  TRNInput/1 -> Bus Selector1/1
  Bus Selector1/3 -> altINS/1  "<Altitude_INS>"
  Bus Selector1/5 -> GPSDataNotValid/1  "<GPSDataNotValid>"
  Bus Selector1/6 -> Degrees to Radians1/1  "<Latitude_GPS>"
  Bus Selector1/7 -> Degrees to Radians2/1  "<Longitude_GPS>"
  Bus Selector1/8 -> altGPS/1  "<Altitude_GPS>"
  Degrees to Radians2/1 -> lonGPS/1
  Degrees to Radians1/1 -> latGPS/1
  Bus Selector1/10 -> FigureofMerit/1  "<FigureofMerit>"

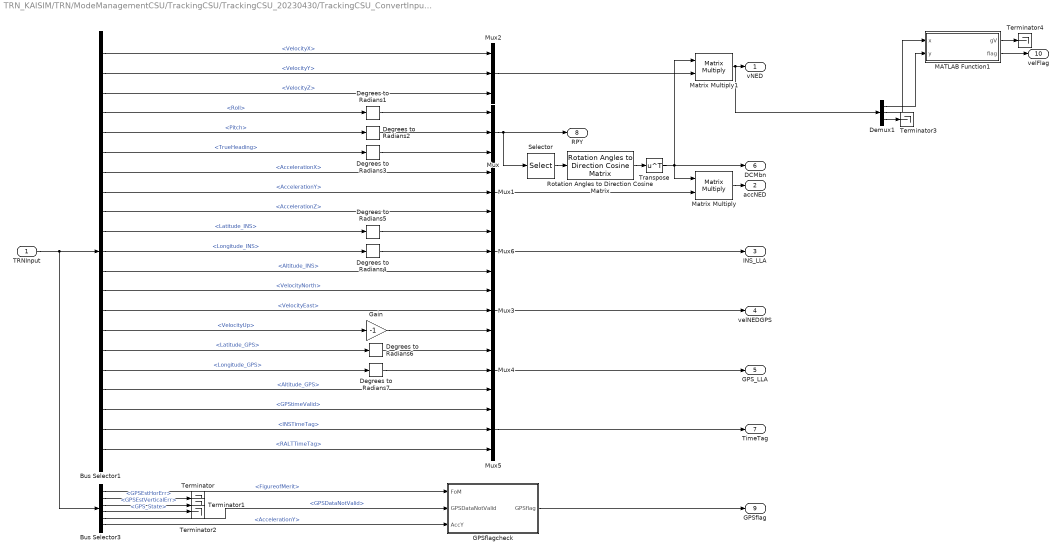
== system TRN_KAISIM/TRN/ModeManagementCSU/TrackingCSU/TrackingCSU_20230430/TrackingCSU_ConvertInput1 ==
  TRNInput : Inport
  Bus Selector1 : BusSelector  OutputSignals=VelocityX,VelocityY,VelocityZ,Roll,Pitch,TrueHeading,AccelerationX,AccelerationY,AccelerationZ,Latitude_INS,Longitude_INS,Altitude_INS,VelocityNorth,VelocityEast,VelocityUp,Latitude_GPS,Longitude_GPS,Altitude_GPS,GPStimeValid,INSTimeTag,RALTTimeTag
  Bus Selector3 : BusSelector  OutputSignals=FigureofMerit,GPSEstHorErr,GPSEstVerticalErr,GPS_State,GPSDataNotValid,AccelerationY
  Degrees to Radians{1..7} (7 alike) : simulink_extras/Transformations/Degrees to Radians
  Demux1 : Demux  Outputs=3
  GPSflagcheck : MATLAB Function  TreatAsAtomicUnit=on
      settings: RTWSystemCode=Nonreusable function  RTWFcnNameOpts=Use subsystem name
  Gain : Gain  Gain=-1
  MATLAB Function1 : MATLAB Function  TreatAsAtomicUnit=on
  Matrix Multiply : Product  Multiplication=Matrix(*)
  Matrix Multiply1 : Product  Multiplication=Matrix(*)
  Mux{,1..6} (7 alike) : Mux  Inputs=3
  Rotation Angles to Direction Cosine Matrix : sharedtransform/Rotation Angles to Direction Cosine Matrix  rotationOrder=ZYX  aMode=aMode
      settings: SourceProductBaseCode=AE,PW,DR,MT,VE
  Selector : Selector  InputPortWidth=3  IndexOptions=Index vector (dialog)  Indices=[3 2 1]  OutputSizes=1
  Terminator{,1..4} (5 alike) : Terminator
  Transpose : Math  Operator=transpose  SignedPower=on
  vNED : Outport  VectorParamsAs1DForOutWhenUnconnected=off
  accNED : Outport  Port=2  VectorParamsAs1DForOutWhenUnconnected=off
  INS_LLA : Outport  Port=3  VectorParamsAs1DForOutWhenUnconnected=off
  velNEDGPS : Outport  Port=4  VectorParamsAs1DForOutWhenUnconnected=off
  GPS_LLA : Outport  Port=5
  DCMbn : Outport  Port=6  VectorParamsAs1DForOutWhenUnconnected=off
  TimeTag : Outport  Port=7  VectorParamsAs1DForOutWhenUnconnected=off
  RPY : Outport  Port=8  VectorParamsAs1DForOutWhenUnconnected=off
  GPSflag : Outport  Port=9  VectorParamsAs1DForOutWhenUnconnected=off
  velFlag : Outport  Port=10  VectorParamsAs1DForOutWhenUnconnected=off
  wires:
  Bus Selector1/18 -> Mux4/3  "<Altitude_GPS>"
  Bus Selector1/17 -> Degrees to Radians7/1  "<Longitude_GPS>"
  Degrees to Radians7/1 -> Mux4/2
  Bus Selector1/21 -> Mux5/3  "<RALTTimeTag>"
  Bus Selector1/20 -> Mux5/2  "<INSTimeTag>"
  Bus Selector1/19 -> Mux5/1  "<GPStimeValid>"
  Gain/1 -> Mux3/3
  Bus Selector1/15 -> Gain/1  "<VelocityUp>"
  Bus Selector1/14 -> Mux3/2  "<VelocityEast>"
  Bus Selector1/13 -> Mux3/1  "<VelocityNorth>"
  Bus Selector1/3 -> Mux2/3  "<VelocityZ>"
  Bus Selector1/1 -> Mux2/1  "<VelocityX>"
  Bus Selector1/4 -> Degrees to Radians1/1  "<Roll>"
  Bus Selector1/2 -> Mux2/2  "<VelocityY>"
  TRNInput/1 -> Bus Selector3/1, Bus Selector1/1
  Bus Selector1/6 -> Degrees to Radians3/1  "<TrueHeading>"
  Degrees to Radians2/1 -> Mux/2
  Degrees to Radians3/1 -> Mux/3
  Mux/1 -> Selector/1, RPY/1
  Bus Selector1/7 -> Mux1/1  "<AccelerationX>"
  Bus Selector1/5 -> Degrees to Radians2/1  "<Pitch>"
  Degrees to Radians1/1 -> Mux/1
  Bus Selector1/9 -> Mux1/3  "<AccelerationZ>"
  Bus Selector1/8 -> Mux1/2  "<AccelerationY>"
  Matrix Multiply1/1 -> Demux1/1, vNED/1
  Matrix Multiply/1 -> accNED/1
  Mux1/1 -> Matrix Multiply/2
  Bus Selector1/10 -> Degrees to Radians5/1  "<Latitude_INS>"
  Transpose/1 -> Matrix Multiply/1, DCMbn/1, Matrix Multiply1/1
  Mux2/1 -> Matrix Multiply1/2
  Rotation Angles to Direction Cosine Matrix/1 -> Transpose/1
  Bus Selector1/11 -> Degrees to Radians4/1  "<Longitude_INS>"
  Degrees to Radians6/1 -> Mux4/1
  Bus Selector1/16 -> Degrees to Radians6/1  "<Latitude_GPS>"
  Selector/1 -> Rotation Angles to Direction Cosine Matrix/1
  Bus Selector3/5 -> GPSflagcheck/2(GPSDataNotValid)  "<GPSDataNotValid>"
  Mux4/1 -> GPS_LLA/1
  Mux3/1 -> velNEDGPS/1
  GPSflagcheck/1(GPSflag) -> GPSflag/1
  Bus Selector3/6 -> GPSflagcheck/3(AccY)  "<AccelerationY>"
  Mux5/1 -> TimeTag/1
  Degrees to Radians5/1 -> Mux6/1
  Degrees to Radians4/1 -> Mux6/2
  Bus Selector1/12 -> Mux6/3  "<Altitude_INS>"
  Mux6/1 -> INS_LLA/1
  Bus Selector3/1 -> GPSflagcheck/1(FoM)  "<FigureofMerit>"
  Demux1/1 -> MATLAB Function1/2(y)
  Demux1/2 -> MATLAB Function1/1(x)
  MATLAB Function1/2(flag) -> velFlag/1
  Bus Selector3/2 -> Terminator/1  "<GPSEstHorErr>"
  Bus Selector3/3 -> Terminator1/1  "<GPSEstVerticalErr>"
  Bus Selector3/4 -> Terminator2/1  "<GPS_State>"
  Demux1/3 -> Terminator3/1
  MATLAB Function1/1(gV) -> Terminator4/1

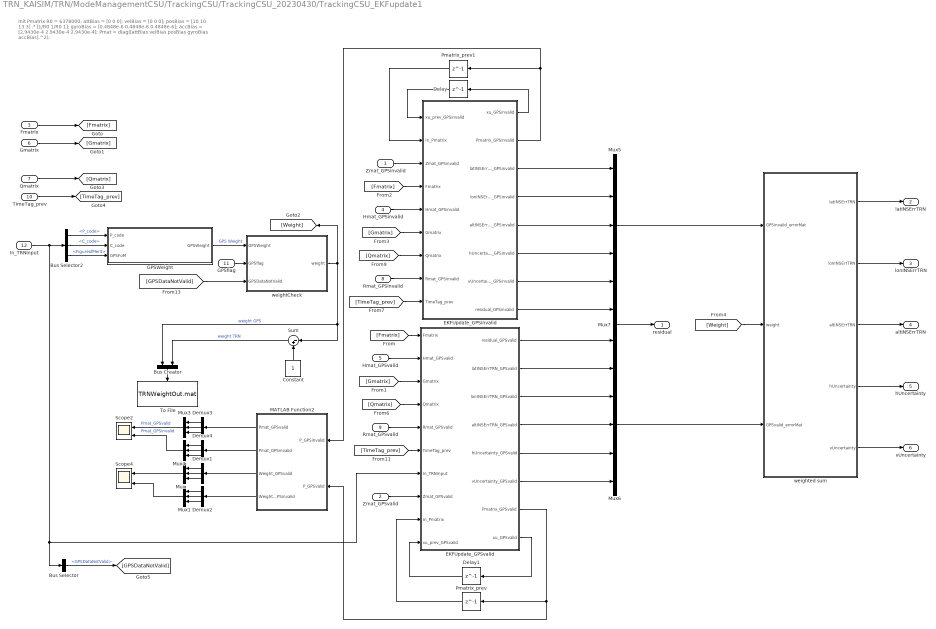
== system TRN_KAISIM/TRN/ModeManagementCSU/TrackingCSU/TrackingCSU_20230430/TrackingCSU_EKFupdate1 ==
  note: Init Pmatrix
      |
      | R0 = 6378000;
      |
      | attBias = [0 0 0];
      | velBias = [0 0 0];
      | posBias = [10 10 13.3] .* [1/R0 1/R0 1];
      | gyroBias = [0.4848e-6 0.4848e-6 0.4848e-6];
      | accBias = [2.9430e-4 2.9430e-4 2.9430e-4];
      |
      | Pmat = diag([attBias velBias posBias gyroBias accBias].^2);
  Zmat_GPSinvalid : Inport  OutDataTypeStr=double  PortDimensions=1
  Zmat_GPSvalid : Inport  Port=2  OutDataTypeStr=double  PortDimensions=[6 1]
  Fmatrix : Inport  Port=3  OutDataTypeStr=double  PortDimensions=[15 15]
  Hmat_GPSinvalid : Inport  Port=4  OutDataTypeStr=double  PortDimensions=[1 15]
  Hmat_GPSvalid : Inport  Port=5  OutDataTypeStr=double  PortDimensions=[6 15]
  Gmatrix : Inport  Port=6  OutDataTypeStr=double  PortDimensions=[15 6]
  Qmatrix : Inport  Port=7  OutDataTypeStr=double  PortDimensions=[6 6]
  Rmat_GPSinvalid : Inport  Port=8  OutDataTypeStr=double  PortDimensions=1
  Rmat_GPSvalid : Inport  Port=9  OutDataTypeStr=double  PortDimensions=[6 6]
  TimeTag_prev : Inport  Port=10
  GPSflag : Inport  Port=11  OutDataTypeStr=uint32  PortDimensions=1
  In_TRNInput : Inport  Port=12  OutDataTypeStr=Bus: TRNInput  PortDimensions=1
  Bus Creator : BusCreator  Inputs=2
  Bus Selector : BusSelector  OutputSignals=GPSDataNotValid
  Bus Selector2 : BusSelector  OutputSignals=P_code,C_code,FigureofMerit
  Constant : Constant
  Delay : Delay  DelayLength=1  InitialCondition=[0.0; 0.0; 0.0; 0.0; 0.0; 0.0; 0.0; 0.0; 0.0; 0.0; 0.0; 0.0; 0.0; 0.0; 0.0]
  Delay1 : Delay  DelayLength=1  InitialCondition=[0.0; 0.0; 0.0; 0.0; 0.0; 0.0; 0.0; 0.0; 0.0; 0.0; 0.0; 0.0; 0.0; 0.0; 0.0]
  Demux{1..4} (4 alike) : Demux  Outputs=3
  EKFUpdate_GPSinvalid : Subsystem  TreatAsAtomicUnit=on
      settings: RTWSystemCode=Nonreusable function  RTWFcnNameOpts=Use subsystem name
  EKFUpdate_GPSvalid : Subsystem  TreatAsAtomicUnit=on
      settings: RTWSystemCode=Nonreusable function  RTWFcnNameOpts=Use subsystem name
  GPSWeight : MATLAB Function  TreatAsAtomicUnit=on
  MATLAB Function2 : MATLAB Function  TreatAsAtomicUnit=on
  Mux{,1,3..4} (4 alike) : Mux  Inputs=3
  Mux5 : Mux  Inputs=5
  Mux6 : Mux  Inputs=5
  Mux7 : Mux  Inputs=2
  Pmatrix_prev : Delay  DelayLength=1  InitialCondition="diag([0 0 0 0 0 0  10/6378000 10/6378000 13.3 0.0 0.0 0.0 0.00014 0.00014 0.00014 ].^2);"
  Pmatrix_prev1 : Delay  DelayLength=1  InitialCondition="diag([0 0 0 0 0 0  10/6378000 10/6378000 13.3 0.0 0.0 0.0 0.00014 0.00014 0.00014 ].^2);"
  Scope2 : Scope  NumInputPorts=2
  Scope4 : Scope  NumInputPorts=2
  Sum : Sum  Inputs=|-+
  To File : ToFile  Filename=TRNWeightOut.mat  MatrixName=Out_TRNWeight  SaveFormat=Timeseries
  weightCheck : MATLAB Function  TreatAsAtomicUnit=on
  weighted sum : MATLAB Function  TreatAsAtomicUnit=on
  residual : Outport
  latINSErrTRN : Outport  Port=2
  lonINSErrTRN : Outport  Port=3
  altINSErrTRN : Outport  Port=4
  hUncertainty : Outport  Port=5
  vUncertainty : Outport  Port=6
  wires:
  weighted sum/5(vUncertainty) -> vUncertainty/1
  [Gmatrix] -> EKFUpdate_GPSvalid/3(Gmatrix)
  [Qmatrix] -> EKFUpdate_GPSvalid/4(Qmatrix)
  Rmat_GPSinvalid/1 -> EKFUpdate_GPSinvalid/8(Rmat_GPSinvalid)
  Hmat_GPSvalid/1 -> EKFUpdate_GPSvalid/2(Hmat_GPSvalid)
  Zmat_GPSvalid/1 -> EKFUpdate_GPSvalid/8(Zmat_GPSvalid)
  In_TRNInput/1 -> Bus Selector/1, EKFUpdate_GPSvalid/7(In_TRNInput), Bus Selector2/1
  Hmat_GPSinvalid/1 -> EKFUpdate_GPSinvalid/5(Hmat_GPSinvalid)
  weighted sum/1(latINSErrTRN) -> latINSErrTRN/1
  [Fmatrix] -> EKFUpdate_GPSinvalid/4(Fmatrix)
  Qmatrix/1 -> [Qmatrix]
  Gmatrix/1 -> [Gmatrix]
  weighted sum/2(lonINSErrTRN) -> lonINSErrTRN/1
  Fmatrix/1 -> [Fmatrix]
  [Fmatrix] -> EKFUpdate_GPSvalid/1(Fmatrix)
  weighted sum/3(altINSErrTRN) -> altINSErrTRN/1
  Rmat_GPSvalid/1 -> EKFUpdate_GPSvalid/5(Rmat_GPSvalid)
  weighted sum/4(hUncertainty) -> hUncertainty/1
  Zmat_GPSinvalid/1 -> EKFUpdate_GPSinvalid/3(Zmat_GPSinvalid)
  [Qmatrix] -> EKFUpdate_GPSinvalid/7(Qmatrix)
  Bus Selector/1 -> [GPSDataNotValid]  "<GPSDataNotValid>"
  [Gmatrix] -> EKFUpdate_GPSinvalid/6(Gmatrix)
  TimeTag_prev/1 -> [TimeTag_prev]
  [TimeTag_prev] -> EKFUpdate_GPSinvalid/9(TimeTag_prev)
  EKFUpdate_GPSinvalid/1(xu_GPSinvalid) -> Delay/1
  [TimeTag_prev] -> EKFUpdate_GPSvalid/6(TimeTag_prev)
  EKFUpdate_GPSvalid/8(xu_GPSvalid) -> Delay1/1
  Bus Selector2/1 -> GPSWeight/1(P_code)  "<P_code>"
  Bus Selector2/3 -> GPSWeight/3(GPSFoM)  "<FigureofMerit>"
  GPSflag/1 -> weightCheck/2(GPSflag)
  [GPSDataNotValid] -> weightCheck/3(GPSDataNotValid)
  MATLAB Function2/3(Weight_GPSvalid) -> Demux1/1
  MATLAB Function2/4(Weight_GPSinvalid) -> Demux2/1
  Demux1/2 -> Mux/2
  Demux1/1 -> Mux/1
  Demux1/3 -> Mux/3
  Mux/1 -> Scope4/1
  Demux2/2 -> Mux1/2
  Demux2/1 -> Mux1/1
  Demux2/3 -> Mux1/3
  Mux1/1 -> Scope4/2
  Bus Selector2/2 -> GPSWeight/2(C_code)  "<C_code>"
  Sum/1 -> Bus Creator/2  "weight TRN"
  weightCheck/1(weight) -> [Weight], Bus Creator/1, Sum/1  "weight GPS"
  GPSWeight/1(GPSWeight) -> weightCheck/1(GPSWeight)  "GPS Weight"
  Demux3/3 -> Mux3/3
  MATLAB Function2/2(Pmat_GPSinvalid) -> Demux4/1
  Mux3/1 -> Scope2/1  "Pmat_GPSvalid"
  Mux4/1 -> Scope2/2  "Pmat_GPSinvalid"
  Demux3/1 -> Mux3/1
  Demux4/1 -> Mux4/1
  Demux3/2 -> Mux3/2
  Demux4/2 -> Mux4/2
  MATLAB Function2/1(Pmat_GPSvalid) -> Demux3/1
  Demux4/3 -> Mux4/3
  Constant/1 -> Sum/2
  EKFUpdate_GPSvalid/7(Pmatrix_GPSvalid) -> MATLAB Function2/2(P_GPSvalid), Pmatrix_prev/1
  EKFUpdate_GPSinvalid/2(Pmatrix_GPSinvalid) -> Pmatrix_prev1/1, MATLAB Function2/1(P_GPSinvalid)
  EKFUpdate_GPSinvalid/3(latINSErrTRN_GPSinvalid) -> Mux5/1
  EKFUpdate_GPSinvalid/4(lonINSErrTRN_GPSinvalid) -> Mux5/2
  EKFUpdate_GPSinvalid/5(altINSErrTRN_GPSinvalid) -> Mux5/3
  EKFUpdate_GPSinvalid/6(hUncertainty_GPSinvalid) -> Mux5/4
  EKFUpdate_GPSinvalid/7(vUncertainty_GPSinvalid) -> Mux5/5
  EKFUpdate_GPSvalid/2(latINSErrTRN_GPSvalid) -> Mux6/1
  EKFUpdate_GPSvalid/3(lonINSErrTRN_GPSvalid) -> Mux6/2
  EKFUpdate_GPSvalid/4(altINSErrTRN_GPSvalid) -> Mux6/3
  EKFUpdate_GPSvalid/5(hUncertainty_GPSvalid) -> Mux6/4
  EKFUpdate_GPSvalid/6(vUncertainty_GPSvalid) -> Mux6/5
  Delay/1 -> EKFUpdate_GPSinvalid/1(xu_prev_GPSinvalid)
  Delay1/1 -> EKFUpdate_GPSvalid/10(xu_prev_GPSvalid)
  Mux7/1 -> residual/1
  EKFUpdate_GPSinvalid/8(residual_GPSinvalid) -> Mux7/1
  EKFUpdate_GPSvalid/1(residual_GPSvalid) -> Mux7/2
  Pmatrix_prev1/1 -> EKFUpdate_GPSinvalid/2(In_Pmatrix)
  Pmatrix_prev/1 -> EKFUpdate_GPSvalid/9(In_Pmatrix)
  Mux5/1 -> weighted sum/1(GPSinvalid_errorMat)
  Mux6/1 -> weighted sum/3(GPSvalid_errorMat)
  [Weight] -> weighted sum/2(weight)
  Bus Creator/1 -> To File/1

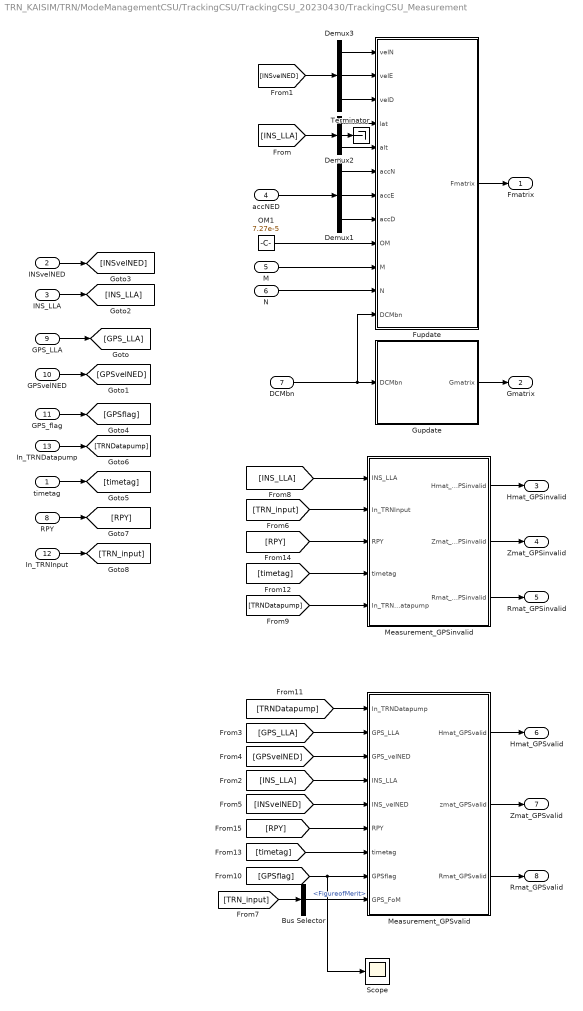
== system TRN_KAISIM/TRN/ModeManagementCSU/TrackingCSU/TrackingCSU_20230430/TrackingCSU_Measurement ==
  timetag : Inport
  INSvelNED : Inport  Port=2
  INS_LLA : Inport  Port=3
  accNED : Inport  Port=4
  M : Inport  Port=5
  N : Inport  Port=6
  DCMbn : Inport  Port=7
  RPY : Inport  Port=8
  GPS_LLA : Inport  Port=9
  GPSvelNED : Inport  Port=10
  GPS_flag : Inport  Port=11
  In_TRNInput : Inport  Port=12
  In_TRNDatapump : Inport  Port=13
  Bus Selector : BusSelector  OutputSignals=FigureofMerit
  Demux1 : Demux  Outputs=3
  Demux2 : Demux  Outputs=3
  Demux3 : Demux  Outputs=3
  Fupdate : MATLAB Function  TreatAsAtomicUnit=on
      settings: RTWSystemCode=Nonreusable function  RTWFcnNameOpts=Use subsystem name
  Gupdate : MATLAB Function  TreatAsAtomicUnit=on
      settings: RTWSystemCode=Nonreusable function  RTWFcnNameOpts=Use subsystem name
  Measurement_GPSinvalid : Subsystem  TreatAsAtomicUnit=on
      settings: RTWSystemCode=Nonreusable function  RTWFcnNameOpts=Use subsystem name
  Measurement_GPSvalid : Subsystem  TreatAsAtomicUnit=on
      settings: RTWSystemCode=Nonreusable function  RTWFcnNameOpts=Use subsystem name
  OM1 : Constant  Value=7.27e-5
  Scope : Scope
  Terminator : Terminator
  Fmatrix : Outport
  Gmatrix : Outport  Port=2
  Hmat_GPSinvalid : Outport  Port=3
  Zmat_GPSinvalid : Outport  Port=4
  Rmat_GPSinvalid : Outport  Port=5
  Hmat_GPSvalid : Outport  Port=6
  Zmat_GPSvalid : Outport  Port=7
  Rmat_GPSvalid : Outport  Port=8
  wires:
  [TRN_input] -> Measurement_GPSinvalid/2(In_TRNInput)
  In_TRNInput/1 -> [TRN_input]
  Measurement_GPSvalid/3(Rmat_GPSvalid) -> Rmat_GPSvalid/1
  Measurement_GPSvalid/2(zmat_GPSvalid) -> Zmat_GPSvalid/1
  Measurement_GPSvalid/1(Hmat_GPSvalid) -> Hmat_GPSvalid/1
  Measurement_GPSinvalid/3(Rmat_GPSinvalid) -> Rmat_GPSinvalid/1
  Measurement_GPSinvalid/2(Zmat_GPSinvalid) -> Zmat_GPSinvalid/1
  Measurement_GPSinvalid/1(Hmat_GPSinvalid) -> Hmat_GPSinvalid/1
  [RPY] -> Measurement_GPSvalid/6(RPY)
  [RPY] -> Measurement_GPSinvalid/3(RPY)
  RPY/1 -> [RPY]
  [timetag] -> Measurement_GPSvalid/7(timetag)
  [timetag] -> Measurement_GPSinvalid/4(timetag)
  [TRNDatapump] -> Measurement_GPSinvalid/5(In_TRNDatapump)
  In_TRNDatapump/1 -> [TRNDatapump]
  timetag/1 -> [timetag]
  [INSvelNED] -> Measurement_GPSvalid/5(INS_velNED)
  [INS_LLA] -> Measurement_GPSvalid/4(INS_LLA)
  [GPSvelNED] -> Measurement_GPSvalid/3(GPS_velNED)
  [GPS_LLA] -> Measurement_GPSvalid/2(GPS_LLA)
  [GPSflag] -> Measurement_GPSvalid/8(GPSflag), Scope/1
  GPS_flag/1 -> [GPSflag]
  [INS_LLA] -> Measurement_GPSinvalid/1(INS_LLA)
  [INSvelNED] -> Demux3/1
  [INS_LLA] -> Demux2/1
  Gupdate/1(Gmatrix) -> Gmatrix/1
  INSvelNED/1 -> [INSvelNED]
  INS_LLA/1 -> [INS_LLA]
  GPSvelNED/1 -> [GPSvelNED]
  GPS_LLA/1 -> [GPS_LLA]
  Demux2/3 -> Fupdate/5(alt)
  Demux2/1 -> Fupdate/4(lat)
  M/1 -> Fupdate/10(M)
  accNED/1 -> Demux1/1
  N/1 -> Fupdate/11(N)
  DCMbn/1 -> Fupdate/12(DCMbn), Gupdate/1(DCMbn)
  Fupdate/1(Fmatrix) -> Fmatrix/1
  Demux1/1 -> Fupdate/6(accN)
  Demux3/2 -> Fupdate/2(velE)
  Demux3/3 -> Fupdate/3(velD)
  Demux1/2 -> Fupdate/7(accE)
  Demux3/1 -> Fupdate/1(velN)
  OM1/1 -> Fupdate/9(OM)
  Demux1/3 -> Fupdate/8(accD)
  [TRN_input] -> Bus Selector/1
  Bus Selector/1 -> Measurement_GPSvalid/9(GPS_FoM)  "<FigureofMerit>"
  [TRNDatapump] -> Measurement_GPSvalid/1(In_TRNDatapump)
  Demux2/2 -> Terminator/1

== system TRN_KAISIM/TRN/ModeManagementCSU/TrackingCSU/TrackingCSU_20230430/TrackingCSU_EKFupdate1/EKFUpdate_GPSinvalid ==
  xu_prev_GPSinvalid : Inport
  In_Pmatrix : Inport  Port=2  OutDataTypeStr=double  PortDimensions=[15 15]
  Zmat_GPSinvalid : Inport  Port=3  OutDataTypeStr=double  PortDimensions=1
  Fmatrix : Inport  Port=4  OutDataTypeStr=double  PortDimensions=[15 15]
  Hmat_GPSinvalid : Inport  Port=5  OutDataTypeStr=double  PortDimensions=[1 15]
  Gmatrix : Inport  Port=6  OutDataTypeStr=double  PortDimensions=[15 6]
  Qmatrix : Inport  Port=7  OutDataTypeStr=double  PortDimensions=[6 6]
  Rmat_GPSinvalid : Inport  Port=8  OutDataTypeStr=double  PortDimensions=1
  TimeTag_prev : Inport  Port=9
  EKFUpdate_GPSinvalid1 : MATLAB Function  Commented=on  TreatAsAtomicUnit=on
      settings: RTWSystemCode=Nonreusable function  RTWFcnNameOpts=Use subsystem name
  EKFUpdate_Predict_GPSinvalid : MATLAB Function  TreatAsAtomicUnit=on
      settings: RTWSystemCode=Nonreusable function  RTWFcnNameOpts=Use subsystem name
  EKFUpdate_Update_GPSinvalid : MATLAB Function  TreatAsAtomicUnit=on
      settings: RTWSystemCode=Nonreusable function  RTWFcnNameOpts=Use subsystem name
  dt : Constant  Value=0.04  OutDataTypeStr=double
  xu_GPSinvalid : Outport
  Pmatrix_GPSinvalid : Outport  Port=2
  latINSErrTRN_GPSinvalid : Outport  Port=3
  lonINSErrTRN_GPSinvalid : Outport  Port=4
  altINSErrTRN_GPSinvalid : Outport  Port=5
  hUncertainty_GPSinvalid : Outport  Port=6
  vUncertainty_GPSinvalid : Outport  Port=7
  residual_GPSinvalid : Outport  Port=8
  wires:
  EKFUpdate_Predict_GPSinvalid/1(I) -> EKFUpdate_Update_GPSinvalid/1(I)
  EKFUpdate_Update_GPSinvalid/2(P_GPSinvalid) -> Pmatrix_GPSinvalid/1
  EKFUpdate_Update_GPSinvalid/7(vUncertainty_GPSinvalid) -> vUncertainty_GPSinvalid/1
  EKFUpdate_Update_GPSinvalid/6(hUncertainty_GPSinvalid) -> hUncertainty_GPSinvalid/1
  EKFUpdate_Update_GPSinvalid/1(xu_GPSinvalid) -> xu_GPSinvalid/1
  EKFUpdate_Predict_GPSinvalid/2(xp) -> EKFUpdate_Update_GPSinvalid/2(xp)
  EKFUpdate_Predict_GPSinvalid/5(K) -> EKFUpdate_Update_GPSinvalid/4(K)
  EKFUpdate_Update_GPSinvalid/5(altINSErrTRN_GPSinvalid) -> altINSErrTRN_GPSinvalid/1
  EKFUpdate_Update_GPSinvalid/4(lonINSErrTRN_GPSinvalid) -> lonINSErrTRN_GPSinvalid/1
  EKFUpdate_Update_GPSinvalid/3(latINSErrTRN_GPSinvalid) -> latINSErrTRN_GPSinvalid/1
  Qmatrix/1 -> EKFUpdate_Predict_GPSinvalid/6(Q)
  Fmatrix/1 -> EKFUpdate_Predict_GPSinvalid/2(Fmatrix)
  Gmatrix/1 -> EKFUpdate_Predict_GPSinvalid/4(Gmatrix)
  Hmat_GPSinvalid/1 -> EKFUpdate_Predict_GPSinvalid/3(Hmat_GPSinvalid), EKFUpdate_Update_GPSinvalid/6(Hmat_GPSinvalid)
  EKFUpdate_Predict_GPSinvalid/3(Pp) -> EKFUpdate_Update_GPSinvalid/3(Pp)
  dt/1 -> EKFUpdate_Predict_GPSinvalid/8(dt)
  Zmat_GPSinvalid/1 -> EKFUpdate_Predict_GPSinvalid/1(Zmat_GPSinvalid), EKFUpdate_Update_GPSinvalid/5(Zmat_GPSinvalid)
  EKFUpdate_Predict_GPSinvalid/4(residual_GPSinvalid) -> residual_GPSinvalid/1
  In_Pmatrix/1 -> EKFUpdate_Predict_GPSinvalid/5(P)
  Rmat_GPSinvalid/1 -> EKFUpdate_Predict_GPSinvalid/7(Rmat_GPSinvalid), EKFUpdate_Update_GPSinvalid/7(Rmat_GPSinvalid)
  TimeTag_prev/1 -> EKFUpdate_Update_GPSinvalid/9(TimeTag_Prev)
  xu_prev_GPSinvalid/1 -> EKFUpdate_Update_GPSinvalid/8(xu_prev_GPSinvalid)

== system TRN_KAISIM/TRN/ModeManagementCSU/TrackingCSU/TrackingCSU_20230430/TrackingCSU_EKFupdate1/EKFUpdate_GPSvalid ==
  Fmatrix : Inport  OutDataTypeStr=double  PortDimensions=[15 15]
  Hmat_GPSvalid : Inport  Port=2  OutDataTypeStr=double  PortDimensions=[6 15]
  Gmatrix : Inport  Port=3  OutDataTypeStr=double  PortDimensions=[15 6]
  Qmatrix : Inport  Port=4  OutDataTypeStr=double  PortDimensions=[6 6]
  Rmat_GPSvalid : Inport  Port=5  OutDataTypeStr=double  PortDimensions=[6 6]
  TimeTag_prev : Inport  Port=6
  In_TRNInput : Inport  Port=7  OutDataTypeStr=Bus: TRNInput  PortDimensions=1
  Zmat_GPSvalid : Inport  Port=8  OutDataTypeStr=double  PortDimensions=[6 1]
  In_Pmatrix : Inport  Port=9  OutDataTypeStr=double  PortDimensions=[15 15]
  xu_prev_GPSvalid : Inport  Port=10
  Bus Selector2 : BusSelector  OutputSignals=GPSEstHorErr,GPSEstVerticalErr
  EKFUpdate_Kgain_GPSvalid : MATLAB Function  TreatAsAtomicUnit=on
      settings: RTWSystemCode=Nonreusable function  RTWFcnNameOpts=Use subsystem name
  EKFUpdate_Predict_GPSvalid : MATLAB Function  TreatAsAtomicUnit=on
      settings: RTWSystemCode=Nonreusable function  RTWFcnNameOpts=Use subsystem name
  EKFUpdate_Update_GPSvalid : MATLAB Function  TreatAsAtomicUnit=on
      settings: RTWSystemCode=Nonreusable function  RTWFcnNameOpts=Use subsystem name
  dt : Constant  Value=0.04  OutDataTypeStr=double
  residual_GPSvalid : Outport
  latINSErrTRN_GPSvalid : Outport  Port=2
  lonINSErrTRN_GPSvalid : Outport  Port=3
  altINSErrTRN_GPSvalid : Outport  Port=4
  hUncertainty_GPSvalid : Outport  Port=5
  vUncertainty_GPSvalid : Outport  Port=6
  Pmatrix_GPSvalid : Outport  Port=7
  xu_GPSvalid : Outport  Port=8
  wires:
  EKFUpdate_Predict_GPSvalid/4(residual_GPSvalid) -> residual_GPSvalid/1
  EKFUpdate_Kgain_GPSvalid/1(K) -> EKFUpdate_Update_GPSvalid/4(K)
  EKFUpdate_Predict_GPSvalid/1(I) -> EKFUpdate_Update_GPSvalid/1(I)
  EKFUpdate_Predict_GPSvalid/3(Pp) -> EKFUpdate_Update_GPSvalid/3(Pp), EKFUpdate_Kgain_GPSvalid/3(Pp)
  EKFUpdate_Predict_GPSvalid/2(xp) -> EKFUpdate_Update_GPSvalid/2(xp)
  EKFUpdate_Update_GPSvalid/1(xu_GPSvalid) -> xu_GPSvalid/1
  EKFUpdate_Update_GPSvalid/7(vUncertainty_GPSvalid) -> vUncertainty_GPSvalid/1
  EKFUpdate_Update_GPSvalid/6(hUncertainty_GPSvalid) -> hUncertainty_GPSvalid/1
  EKFUpdate_Update_GPSvalid/4(lonINSErrTRN_GPSvalid) -> lonINSErrTRN_GPSvalid/1
  EKFUpdate_Update_GPSvalid/2(P_GPSvalid) -> Pmatrix_GPSvalid/1
  EKFUpdate_Update_GPSvalid/5(altINSErrTRN_GPSvalid) -> altINSErrTRN_GPSvalid/1
  EKFUpdate_Update_GPSvalid/3(latINSErrTRN_GPSvalid) -> latINSErrTRN_GPSvalid/1
  Qmatrix/1 -> EKFUpdate_Predict_GPSvalid/4(Q)
  dt/1 -> EKFUpdate_Predict_GPSvalid/5(dt)
  Rmat_GPSvalid/1 -> EKFUpdate_Kgain_GPSvalid/2(Rmat_GPSvalid), EKFUpdate_Update_GPSvalid/7(Rmat_GPSvalid)
  Bus Selector2/1 -> EKFUpdate_Update_GPSvalid/10(GPSHorUncert)  "<GPSEstHorErr>"
  Bus Selector2/2 -> EKFUpdate_Update_GPSvalid/11(GPSVerUncert)  "<GPSEstVerticalErr>"
  In_Pmatrix/1 -> EKFUpdate_Predict_GPSvalid/3(P)
  Gmatrix/1 -> EKFUpdate_Predict_GPSvalid/2(Gmatrix)
  Hmat_GPSvalid/1 -> EKFUpdate_Kgain_GPSvalid/1(Hmat_GPSvalid), EKFUpdate_Update_GPSvalid/6(Hmat_GPSvalid)
  Fmatrix/1 -> EKFUpdate_Predict_GPSvalid/1(Fmatrix)
  Zmat_GPSvalid/1 -> EKFUpdate_Predict_GPSvalid/6(Zmat_GPSvalid), EKFUpdate_Update_GPSvalid/5(Zmat_GPSvalid)
  In_TRNInput/1 -> Bus Selector2/1
  xu_prev_GPSvalid/1 -> EKFUpdate_Update_GPSvalid/8(xu_prev_GPSvalid)
  TimeTag_prev/1 -> EKFUpdate_Update_GPSvalid/9(TimeTag_Prev)

== system TRN_KAISIM/TRN/ModeManagementCSU/TrackingCSU/TrackingCSU_20230430/TrackingCSU_Measurement/Measurement_GPSinvalid ==
  note: Measurement Prameters
      | residualValid : True[Update] / False[INS propagation]
      | Result_Prev[1] : False[Update] / True[INS propagation]
  INS_LLA : Inport
  In_TRNInput : Inport  Port=2
  RPY : Inport  Port=3
  timetag : Inport  Port=4
  In_TRNDatapump : Inport  Port=5
  AND : Logic  IconShape=distinctive  AllPortsSameDT=off  OutDataTypeStr=boolean
  Bus Selector : BusSelector  OutputSignals=Result_Prev
  Bus Selector1 : BusSelector  OutputSignals=RALTAltitude
  Bus Selector2 : BusSelector  OutputSignals=RALTValid
  Data Store Read1 : DataStoreRead  DataStoreName=RES  IndexOptions=Index vector (dialog)  Indices=1  OutputSizes=1
  Data Type Conversion : DataTypeConversion  OutDataTypeStr=boolean  SaturateOnIntegerOverflow=off  RndMeth=Floor
  Data Type Conversion1 : DataTypeConversion  OutDataTypeStr=int32  SaturateOnIntegerOverflow=off  RndMeth=Floor
  Delay : Delay  DelayLength=1  InitialConditionSource=Input port
      settings: InputPortMap=u0,p4
  Demux : Demux  Outputs=6
  Demux10 : Demux  Outputs=3
  Demux4 : Demux  Outputs=3
  Demux5 : Demux  Outputs=3
  MATLAB Function : MATLAB Function  TreatAsAtomicUnit=on
  MesurementUpdate_GPSinvalid : MATLAB Function  TreatAsAtomicUnit=on
      settings: RTWSystemCode=Nonreusable function  RTWFcnNameOpts=Use subsystem name
  MesurementValid_GPSinvalid : MATLAB Function  TreatAsAtomicUnit=on
      settings: RTWSystemCode=Nonreusable function  RTWFcnNameOpts=Use subsystem name
  Mux : Mux  Inputs=5
  Mux1 : Mux  Inputs=2
  Radians to Degrees : simulink_extras/Transformations/Radians to Degrees
  Terminator : Terminator
  Terminator1 : Terminator
  Terminator3 : Terminator
  residualValidCheck : Subsystem
  Hmat_GPSinvalid : Outport
  Zmat_GPSinvalid : Outport  Port=2
  Rmat_GPSinvalid : Outport  Port=3
  wires:
  Radians to Degrees/1 -> MesurementUpdate_GPSinvalid/5(resolution)
  Mux1/1 -> Terminator1/1
  Demux5/2 -> Mux1/2
  Demux5/1 -> Mux1/1
  Mux/1 -> Terminator3/1
  Demux/6 -> Mux/5
  Demux/5 -> Mux/4
  Demux/4 -> Mux/3
  Demux/3 -> Mux/2
  Demux/2 -> Mux/1
  AND/1 -> MesurementValid_GPSinvalid/1(updateValid)
  Data Type Conversion/1 -> AND/2
  Demux/1 -> Data Type Conversion/1
  Bus Selector/1 -> Demux/1  "<Result_Prev>"
  Data Store Read1/1 -> Radians to Degrees/1
  MATLAB Function/1(Rmat) -> Rmat_GPSinvalid/1
  MesurementUpdate_GPSinvalid/2(Zmat_GPSinvalid) -> MesurementValid_GPSinvalid/4(zmat_in)
  In_TRNDatapump/1 -> Bus Selector/1, residualValidCheck/1(TRNDatapump)
  RPY/1 -> Demux4/1
  Delay/1 -> MesurementValid_GPSinvalid/6(RALTTimeTag_temp)
  MesurementValid_GPSinvalid/1(zmat_out) -> Zmat_GPSinvalid/1
  Demux4/2 -> MesurementValid_GPSinvalid/3(pitch)
  residualValidCheck/1(residualValid) -> AND/1
  Data Type Conversion1/1 -> Delay/1, Delay/2, MesurementValid_GPSinvalid/5(RALTTimeTag)
  timetag/1 -> Demux5/1
  Demux4/1 -> MesurementValid_GPSinvalid/2(roll)
  Bus Selector2/1 -> MesurementValid_GPSinvalid/7(RLATvalid)  "<RALTValid>"
  Demux4/3 -> Terminator/1
  MesurementUpdate_GPSinvalid/1(Hmat_GPSinvalid) -> Hmat_GPSinvalid/1
  In_TRNInput/1 -> Bus Selector1/1, Bus Selector2/1
  INS_LLA/1 -> Demux10/1
  Demux10/2 -> MesurementUpdate_GPSinvalid/2(lon)
  Demux10/1 -> MesurementUpdate_GPSinvalid/1(lat)
  Bus Selector1/1 -> MesurementUpdate_GPSinvalid/4(RALTAltitude)  "<RALTAltitude>"
  Demux10/3 -> MesurementUpdate_GPSinvalid/3(alt)
  Demux5/3 -> Data Type Conversion1/1
